simulink model "model11"  (R2023b)
settings: Solver=FixedStepAuto  StartTime=0.0  StopTime=10.0  RelTol=1e-3
model workspace (MAT data in the model file):
  c1 = 100
settings Model: Creator=z004f2se  LastModifiedBy=z004f2se

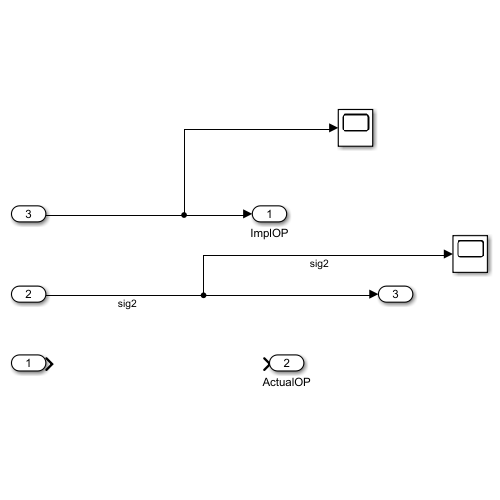
[thumbnail: Simulink's stored preview of the top-level diagram]
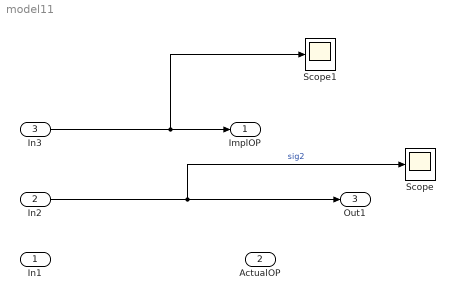
== system model11 ==
  In1 : Inport
  In2 : Inport  Port=2
  In3 : Inport  Port=3
  Scope : Scope
  Scope1 : Scope
  ImplOP : Outport
  ActualOP : Outport  Port=2
  Out1 : Outport  Port=3
  wires:
  In2/1 -> Scope/1, Out1/1  "sig2"
  In3/1 -> ImplOP/1, Scope1/1
